simulink model "reaction_pendulum"  (R2021b)
settings: Solver=FixedStepDiscrete  StartTime=0.0  StopTime=140  FixedStep=h  RelTol=1e-3  EnableMultiTasking=on
PreLoadFcn:
  | warning('off','MATLAB:dispatcher:InexactMatch');
InitFcn:
  | hwinit
values from neighbouring files (symbols this model uses):
  h = 0.05    [Identified_system1_data.mat]    (also in Identified_system2_data.mat; Identified_system3_data.mat; Identified_system4_data.mat; MotorID_data.mat)
  K = Synth_LQR(sys, "Greybox")    [A1masterMain.m]    (also in Controller_LQR.mat = [-0.0224541453394 1.5413407747e-07 0.00117109816368 -2.28642; kalman.m = P_1 * H'/(H*P_1*H' + R))
  K_Unst = Synth_LQR(sysUnst, "Greybox")    [A1masterMain.m]
  params = cell2struct([struct2cell(motorparams);struct2cell(pendparams)],[fieldnames(motorparams);fieldnames(pendparams)],1)    [A1masterMain_Measurements.m]
  sys = ss(sys.A, sys.B, eye(nx), zeros(nx,1), h)    [A1masterMain.m]    (also in A1masterMain_Measurements.m; SysIDgrey_fullParamed.m = ss(Ac,Bc,Cc,Dc); SysIDgrey_motor.m = ss(Ac,Bc,Cc,Dc); SysIDgrey_semiParamed.m = ss(Ac,Bc,Cc,Dc))
undefined symbols (not defined in the file or in its folder): DiscIntNeverNeededParam, Discrete, Hinf, HinfI, HinfUnst, HinfUnstI, Ki, Ki_Unst, sysObserver, Time
libraries: simulink x5, mpclib x5, eeGeneralControl x2, ctrlSharedLib x2, sharedTrackingLibrary x1, eeLuenbergerObserver x1, pid_lib x1
settings Model: SimulationMode=external  ExtModeTrigDuration=100000  Creator=user  LastModifiedBy=saumans
settings DataIOCC: SaveFormat=Array  SignalLoggingSaveFormat=ModelDataLogs  SaveOutput=off  SignalLogging=off  DSMLogging=off  SaveTime=off  ReturnWorkspaceOutputs=off
settings OptimizationCC: ExpressionDepthLimit=2147483647  LifeSpan=inf
settings DebuggingCC: UnderspecifiedInitializationDetection=Classic  MergeDetectMultiDrivingBlocksExec=none  SolverPrmCheckMsg=warning  FcnCallInpInsideContextMsg=warning  StateNameClashWarn=warning  SFUnexpectedBacktrackingDiag=warning  SFNoUnconditionalDefaultTransitionDiag=warning  SFExecutionAtInitializationDiag=none  SFMachineParentedDataDiag=warning  ArithmeticOperatorsInVariantConditions=warning
settings HardwareCC: ProdBitPerPointer=32  ProdBitPerSizeT=32  ProdBitPerPtrDiffT=32  ProdLargestAtomicFloat=None  ProdIntDivRoundTo=Undefined  ProdEndianess=Unspecified  ProdWordSize=32  ProdHWDeviceType=32-bit Generic
settings ModelReferenceCC: PropagateSignalLabelsOutOfModel=off
settings SFSimCC: SimUseLocalCustomCode=off  CustomCodeUndefinedFunction=UseInterfaceOnly
settings RTWCC: Description=rpend RTDAC/USB2 (Visual C/C++)  SystemTargetFile=rtcon_rpend_usb2.tlc  TemplateMakefile=rtcon_rpend_vc_usb2_x64.tmf  RTWUseLocalCustomCode=off
settings CodeAppCC: StateflowObjectComments=on
settings STFCustomTargetCC: ModelReferenceCompliant=off  CombineOutputUpdateFcns=on  MatFileLogging=on  GRTInterface=off  SystemTargetFile=rtcon_rpend_usb2.tlc
settings GRTTargetCC: TargetLangStandard=C89/C90 (ANSI)  ModelReferenceCompliant=off  ParMdlRefBuildCompliant=off  CompOptLevelCompliant=off  ConcurrentExecutionCompliant=off  CPPClassGenCompliant=off  UseToolchainInfoCompliant=off  ExtMode=on  ExtModeMexFile=rtcon_ext_comm
settings ConfigComp: CovMetricSettings=dw  CovSaveCumulativeToWorkspaceVar=on  CovSaveSingleToWorkspaceVar=on  CovExternalEMLEnable=off  CovSFcnEnable=off

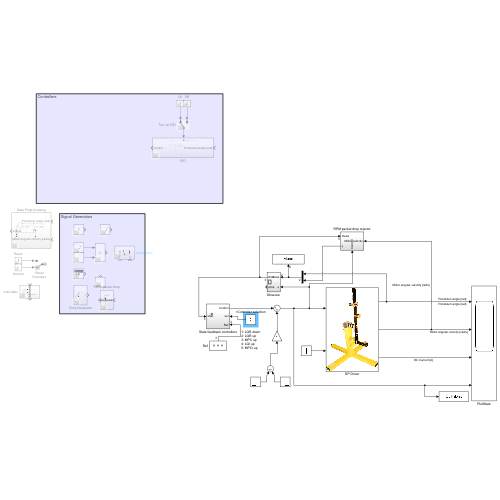
[thumbnail: Simulink's stored preview of the top-level diagram]
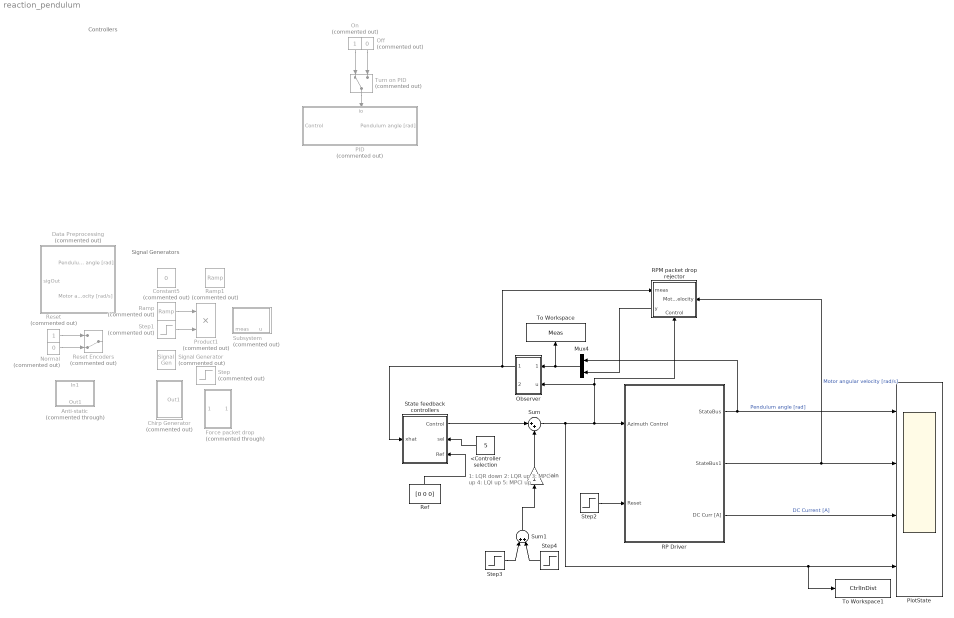
== system reaction_pendulum ==
  note: 1: LQR down
      | 2: LQR up
      | 3: MPC up
      | 4: LQI up
      | 5: MPCI up
  note: Controllers
  note: Signal Generators
  <Controller selection : Constant  Value=5
  Anti-static : Subsystem  Commented=through
  Chirp Generator : Subsystem  Commented=on
  Constant5 : Constant  Commented=on  Value=0
  Data Preprocessing : Subsystem  Commented=on
  Force packet drop : Subsystem  Commented=through
  Gain : Gain
  Mux4 : Mux  Inputs=2
  Normal : Constant  Commented=on  Value=0
  Observer : Subsystem
  Off : Constant  Commented=on  Value=0
  On : Constant  Commented=on
  PID : Subsystem  Commented=on
      settings: PortSchema="{\"entries\":[{\"content\":{\"sides\":[{\"content\":{\"connectorIds\":[\"In1\"]},\"type\":\"ConnectorPlacement.EquallySpacedRectSide\",\"uuid\":\"f2fec2e3-226e-4957-a417-0defdc291ba5\"},{\"content\":{\"connectorIds\":[\"Out1\"],\"side\":\"RIGHT\"},\"type\":\"ConnectorPlacement.EquallySpacedRectSide\",\"uuid\":\"376d4e87-61ea-4bcd-a986-cfc18b67c5cf\"},{\"content\":{\"connectorIds\":[\"In2\"],\"side\":\"TOP\"},\"type\":\"ConnectorPlacement.EquallySpacedRectSide\",\"uuid\":\"5745c80a-bb5a-4df3-811e-7eecb0205f19\"}]},\"type\":\"ConnectorPlacement.EquallySpacedConnector\",\"uuid\":\"e1ac6d12-4a7f-4ceb-9bf6-49805cc7f347\"}],\"packageUris\":[\"http://schema.mathworks.com/mf0/Connector/R2020b\"],\"version\":\"1.0\"}"
  PlotState : Scope  NumInputPorts=4
  Product1 : Product  Commented=on
  RP Driver : Subsystem
      mask Display: image(imread('rwp.JPG'))
  RPM packet drop rejector : Subsystem
      settings: PortSchema="{\"entries\":[{\"content\":{\"sides\":[{\"content\":{\"connectorIds\":[\"In1\"]},\"type\":\"ConnectorPlacement.EquallySpacedRectSide\",\"uuid\":\"dc71c52c-be7a-4309-9ef6-de56d2efa973\"},{\"content\":{\"connectorIds\":[\"In3\",\"Out1\"],\"side\":\"RIGHT\"},\"type\":\"ConnectorPlacement.EquallySpacedRectSide\",\"uuid\":\"4ea731d9-e83e-45db-852e-b55f70ff1dcb\"},{\"content\":{\"connectorIds\":[],\"side\":\"TOP\"},\"type\":\"ConnectorPlacement.EquallySpacedRectSide\",\"uuid\":\"11ed21a3-acf9-42d7-b1cb-d4047d3b6345\"},{\"content\":{\"connectorIds\":[\"In2\"],\"side\":\"BOTTOM\"},\"type\":\"ConnectorPlacement.EquallySpacedRectSide\",\"uuid\":\"19313e71-7ed6-479a-97a2-a24af120137a\"}]},\"type\":\"ConnectorPlacement.EquallySpacedConnector\",\"uuid\":\"3af8e27e-d2cb-4c9f-8435-3e2adc15d5d9\"}],\"packageUris\":[\"http://schema.mathworks.com/mf0/Connector/R2020b\"],\"version\":\"1.0\"}"
  Ramp : simulink/Sources/Ramp  Commented=on  slope=0.5/29  start=1  InitialOutput=0
  Ramp1 : simulink/Sources/Ramp  Commented=on  slope=0.5/29  start=1  InitialOutput=0
  Ref : Constant  Value=[0 0 0]
  Reset : Constant  Commented=on
  Reset Encoders : ManualSwitch  Commented=on  CurrentSetting=0
  Signal Generator : SignalGenerator  Commented=on  Amplitude=0.5  Frequency=0.1
  State feedback controllers : Subsystem
      settings: PortSchema="{\"entries\":[{\"content\":{\"sides\":[{\"content\":{\"connectorIds\":[\"In1\"]},\"type\":\"ConnectorPlacement.EquallySpacedRectSide\",\"uuid\":\"50f77728-1820-4c1e-b55e-992377a2ac74\"},{\"content\":{\"connectorIds\":[\"Out1\",\"In2\",\"In3\"],\"side\":\"RIGHT\"},\"type\":\"ConnectorPlacement.EquallySpacedRectSide\",\"uuid\":\"85e2483e-83dd-4c22-9320-33a68cb16c11\"},{\"content\":{\"connectorIds\":[],\"side\":\"TOP\"},\"type\":\"ConnectorPlacement.EquallySpacedRectSide\",\"uuid\":\"96f413ab-f651-4769-ae7d-08868bc0ab5d\"}]},\"type\":\"ConnectorPlacement.EquallySpacedConnector\",\"uuid\":\"cd5e282e-a58c-452a-9f76-0f6edfd53294\"}],\"packageUris\":[\"http://schema.mathworks.com/mf0/Connector/R2020b\"],\"version\":\"1.0\"}"
  Step : Step  Commented=on  Time=1.5  SampleTime=h
  Step1 : Step  Commented=on  Time=30  Before=1  After=0  SampleTime=h
  Step2 : Step  Time=h  Before=1  After=0  SampleTime=0
  Step3 : Step  Time=2  SampleTime=0
  Step4 : Step  Time=2.2  After=-1  SampleTime=0
  Subsystem : Subsystem  Commented=on
  Sum : Sum  Inputs=|++
  Sum1 : Sum  Inputs=|++|
  To Workspace : ToWorkspace  VariableName=Meas  SampleTime=h
      settings: Save2DSignal=2-D array (concatenate along first dimension)
  To Workspace1 : ToWorkspace  VariableName=CtrlInDist  SaveFormat=Structure With Time  SampleTime=h
      settings: Save2DSignal=2-D array (concatenate along first dimension)
  Turn on PID : ManualSwitch  Commented=on
  wires:
  Normal/1 -> Reset Encoders/2
  Reset/1 -> Reset Encoders/1
  Step2/1 -> RP Driver/2(Reset)
  RP Driver/3(DC Curr [A]) -> PlotState/3  "DC Current [A]"
  RP Driver/2(StateBus1) -> RPM packet drop rejector/1(Motor velocity), PlotState/2  "Motor angular velocity [rad/s]"
  RP Driver/1(StateBus) -> PlotState/1, Mux4/1  "Pendulum angle [rad]"
  On/1 -> Turn on PID/1
  Off/1 -> Turn on PID/2
  Turn on PID/1 -> PID/2(io)
  Step1/1 -> Product1/2
  Ramp/1 -> Product1/1
  <Controller selection/1 -> State feedback controllers/2(sel)
  Ref/1 -> State feedback controllers/3(Ref)
  RPM packet drop rejector/1(y) -> Mux4/2
  Mux4/1 -> To Workspace/1, Observer/1(meas)
  Sum/1 -> To Workspace1/1, PlotState/4, RPM packet drop rejector/2(Control), Observer/2(u), RP Driver/1(Azimuth Control)
  Observer/1(xhat) -> State feedback controllers/1(xhat), RPM packet drop rejector/3(meas)
  State feedback controllers/1(Control) -> Sum/1
  Gain/1 -> Sum/2
  Sum1/1 -> Gain/1
  Step3/1 -> Sum1/1
  Step4/1 -> Sum1/2

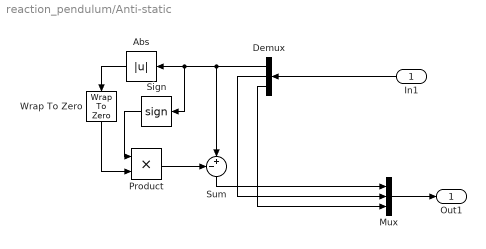
== system reaction_pendulum/Anti-static ==
  In1 : Inport
  Abs : Abs
  Demux : Demux  Outputs=3
  Mux : Mux  Inputs=3
  Product : Product
  Sign : Signum
  Sum : Sum  Inputs=-+|
  Wrap To Zero : simulink/Discontinuities/Wrap To Zero  Threshold=0.005
      settings: SourceProductBaseCode=SL
  Out1 : Outport
  wires:
  Demux/1 -> Sign/1, Abs/1, Sum/2
  Wrap To Zero/1 -> Product/2
  Sum/1 -> Mux/1
  Mux/1 -> Out1/1
  Sign/1 -> Product/1
  Product/1 -> Sum/1
  In1/1 -> Demux/1
  Abs/1 -> Wrap To Zero/1
  Demux/3 -> Mux/3
  Demux/2 -> Mux/2

== system reaction_pendulum/Chirp Generator ==
  Chirp Signal : simulink/Sources/Chirp Signal  f1=0.025  T=100  f2=0.75
  Gain3 : Gain  Gain=0.2
  Product3 : Product
  varMag_chirp_generator : Subsystem
  Out1 : Outport
  wires:
  Gain3/1 -> Out1/1
  Chirp Signal/1 -> Product3/1
  varMag_chirp_generator/1(Out1) -> Product3/2
  Product3/1 -> Gain3/1

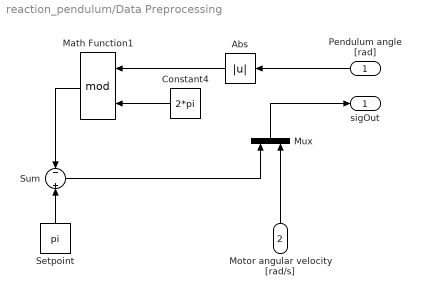
== system reaction_pendulum/Data Preprocessing ==
  Pendulum angle [rad] : Inport
  Motor angular velocity [rad/s] : Inport  Port=2
  Abs : Abs
  Constant4 : Constant  Value=2*pi
  Math Function1 : Math  Operator=mod  SaturateOnIntegerOverflow=on
  Mux : Mux  Inputs=2
  Setpoint : Constant  Value=pi
  Sum : Sum  Inputs=-||+
  sigOut : Outport
  wires:
  Motor angular velocity [rad/s]/1 -> Mux/2
  Sum/1 -> Mux/1
  Abs/1 -> Math Function1/1
  Math Function1/1 -> Sum/1
  Pendulum angle [rad]/1 -> Abs/1
  Setpoint/1 -> Sum/2
  Constant4/1 -> Math Function1/2
  Mux/1 -> sigOut/1

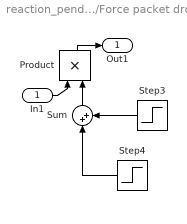
== system reaction_pendulum/Force packet drop ==
  In1 : Inport
  Product : Product
  Step3 : Step  Time=10+7*h  SampleTime=0
  Step4 : Step  Time=10  Before=1  After=0  SampleTime=0
  Sum : Sum  Inputs=|++
  Out1 : Outport
  wires:
  Step4/1 -> Sum/1
  Step3/1 -> Sum/2
  Product/1 -> Out1/1
  Sum/1 -> Product/2
  In1/1 -> Product/1

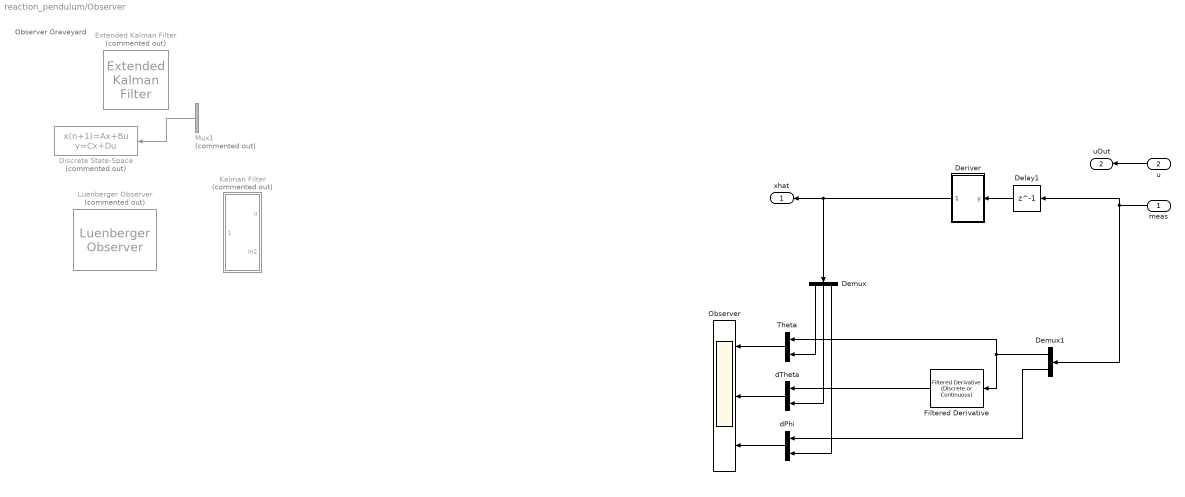
== system reaction_pendulum/Observer ==
  note: Observer Graveyard
  meas : Inport
  u : Inport  Port=2
  Delay1 : Delay  DelayLength=1  InitialCondition=0
  Demux : Demux  Outputs=3
  Demux1 : Demux  Outputs=2
  Deriver : Subsystem
  Discrete State-Space : DiscreteStateSpace  Commented=on  A=sysObserver.A  B=sysObserver.B  C=sysObserver.C  D=sysObserver.D  SampleTime=h
  Extended Kalman Filter : sharedTrackingLibrary/Extended Kalman Filter  Commented=on  StateTransitionFcn=nextIter  HasStateTransitionJacobianFcn=off  HasAdditiveProcessNoise=Additive  ProcessNoise=1  HasTimeVaryingProcessNoise=off  HasStateTransitionFcnExtraArgument=0  InitialState=0  InitialStateCovariance=1  MeasurementFcn1=myMeasurementFcn  HasMeasurementJacobianFcn1=off  HasMeasurementEnablePort1=off  HasAdditiveMeasurementNoise1=Additive  MeasurementNoise1=1  HasTimeVaryingMeasurementNoise1=off  HasMeasurementFcnExtraArgument1=0  MeasurementFcn2=myMeasurementFcn  HasMeasurementJacobianFcn2=off  HasMeasurementEnablePort2=off  HasAdditiveMeasurementNoise2=Additive  MeasurementNoise2=1  HasTimeVaryingMeasurementNoise2=off  HasMeasurementFcnExtraArgument2=0  MeasurementFcn3=myMeasurementFcn  HasMeasurementJacobianFcn3=off  HasMeasurementEnablePort3=off  HasAdditiveMeasurementNoise3=Additive  MeasurementNoise3=1  HasTimeVaryingMeasurementNoise3=off  HasMeasurementFcnExtraArgument3=0  MeasurementFcn4=myMeasurementFcn  HasMeasurementJacobianFcn4=off  HasMeasurementEnablePort4=off  HasAdditiveMeasurementNoise4=Additive  MeasurementNoise4=1  HasTimeVaryingMeasurementNoise4=off  HasMeasurementFcnExtraArgument4=0  MeasurementFcn5=myMeasurementFcn  HasMeasurementJacobianFcn5=off  HasMeasurementEnablePort5=off  HasAdditiveMeasurementNoise5=Additive  MeasurementNoise5=1  HasTimeVaryingMeasurementNoise5=off  HasMeasurementFcnExtraArgument5=0  EnableMultirate=off  StateTransitionFcnSampleTime=1  MeasurementFcn1SampleTime=1  MeasurementFcn2SampleTime=1  MeasurementFcn3SampleTime=1  MeasurementFcn4SampleTime=1  MeasurementFcn5SampleTime=1  UseCurrentEstimator=on  OutputStateCovariance=off  DataType=double  SampleTime=1  NumberOfMeasurements=1
      settings: SourceProductBaseCode=AE,PW,CT,DR,TF,ID,LP,NV,AR,RO,RR,UV,VE
  Filtered Derivative : eeGeneralControl/Filtered Derivative (Discrete or Continuous)  K=1  T=h  B=inf  A=-inf  minRatio=1  init_option=Specify as parameter  x0=0  Ts=h
      settings: SourceProductBaseCode=PS
  Kalman Filter : Subsystem  Commented=on
  Luenberger Observer : eeLuenbergerObserver/Luenberger Observer  Commented=on  StateSpaceType=Discrete-time  Ad=sys.A  Bd=sys.B  Cd=sys.C  Dd=sys.D  A=1  B=1  C=1  D=1  ObserverDesign=Desired eigenvalues  Ld=1  DesiredEigenvalues=0.2+(1:size(sys.A, 2))*0.001  x0=zeros(size(sys.A, 2), 1)  Tsd=0.1  Ts=h
      settings: SourceProductBaseCode=PS
  Mux1 : Mux  Commented=on  Inputs=2
  Observer : Scope  NumInputPorts=3
  Theta : Mux  Inputs=2
  dPhi : Mux  Inputs=2
  dTheta : Mux  Inputs=2
  xhat : Outport
  uOut : Outport  Port=2
  wires:
  meas/1 -> Demux1/1, Delay1/1
  Deriver/1(xhat) -> Demux/1, xhat/1
  Mux1/1 -> Discrete State-Space/1
  Theta/1 -> Observer/1
  dTheta/1 -> Observer/2
  dPhi/1 -> Observer/3
  Filtered Derivative/1 -> dTheta/1
  Demux/1 -> Theta/2
  Demux/2 -> dTheta/2
  Demux/3 -> dPhi/2
  Demux1/1 -> Theta/1, Filtered Derivative/1
  Demux1/2 -> dPhi/1
  u/1 -> uOut/1
  Delay1/1 -> Deriver/1(y)

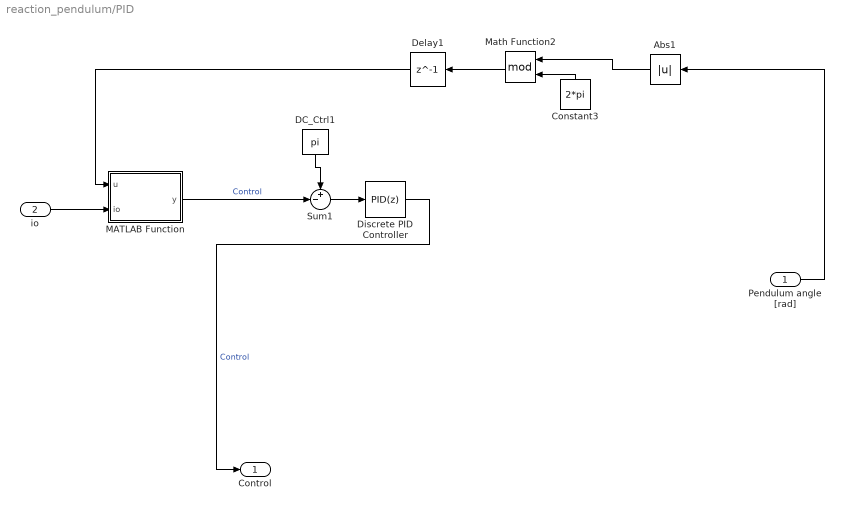
== system reaction_pendulum/PID ==
  Pendulum angle [rad] : Inport
  io : Inport  Port=2
  Abs1 : Abs
  Constant3 : Constant  Value=2*pi
  DC_Ctrl1 : Constant  Value=pi
  Delay1 : Delay  DelayLength=1  InitialCondition=0
  Discrete PID Controller : pid_lib/PID Controller  Controller=PID  Form=Parallel  TimeDomain=Discrete-time  UseExternalTs=off  SampleTime=h  IntegratorMethod=Forward Euler  FilterMethod=Forward Euler  ControllerParametersSource=internal  P=5.451713395638629  I=2.984615384615385  D=2.369230769230769  N=3  UseFilter=on  TunerSelectOption=Frequency Response Based  InitialConditionSource=internal  InitialConditionForIntegrator=0  InitialConditionForFilter=0  DifferentiatorICPrevScaledInput=0  ExternalReset=none  TrackingMode=off  Kt=1  LimitOutput=off  SatLimitsSource=internal  UpperSaturationLimit=inf  LowerSaturationLimit=-inf  LinearizeAsGain=off  AntiWindupMode=none  Kb=1  POutMin=[]  POutMax=[]  IOutMin=[]  IOutMax=[]  DOutMin=[]  DOutMax=[]  NOutMin=[]  NOutMax=[]  SumOutMin=[]  SumOutMax=[]  SaturationOutMin=[]  SaturationOutMax=[]  PParamMin=[]  PParamMax=[]  IParamMin=[]  IParamMax=[]  DParamMin=[]  DParamMax=[]  NParamMin=[]  NParamMax=[]  KbParamMin=[]  KbParamMax=[]  KtParamMin=[]  KtParamMax=[]  KbOutMin=[]  KbOutMax=[]  KtOutMin=[]  KtOutMax=[]  IntegratorOutMin=[]  IntegratorOutMax=[]  FilterOutMin=[]  FilterOutMax=[]  SumI1OutMin=[]  SumI1OutMax=[]  SumI2OutMin=[]  SumI2OutMax=[]  SumI3OutMin=[]  SumI3OutMax=[]  SumI4OutMin=[]  SumI4OutMax=[]  SumDOutMin=[]  SumDOutMax=[]  DifferentiatorOutMin=[]  DifferentiatorOutMax=[]  FilterDiffOutCoefMin=[]  FilterDiffOutCoefMax=[]  ReciprocalOutMin=[]  ReciprocalOutMax=[]  SumDenOutMin=[]  SumDenOutMax=[]  SumNumOutMin=[]  SumNumOutMax=[]  DivideOutMin=[]  DivideOutMax=[]  UdiffTsProdOutMin=[]  UdiffTsProdOutMax=[]  NTsProdOutMin=[]  NTsProdOutMax=[]  UintegralTsProdOutMin=[]  UintegralTsProdOutMax=[]  UngainTsProdOutMin=[]  UngainTsProdOutMax=[]  IntegratorContinuousStateAttributes=''  IntegratorStateMustResolveToSignalObject=off  IntegratorRTWStateStorageClass=Auto  FilterContinuousStateAttributes=''  FilterStateMustResolveToSignalObject=off  FilterRTWStateStorageClass=Auto  ParallelPVariant=InternalParameters  IdealPVariant=Disabled  IVariant=InternalParameters  DVariant=InternalParameters  IntegratorVariant=Discrete  SatVariant=Disabled  AWVariant=Passthrough  PCopyVariant=Disabled  TRVariant=Disabled  FdbkBlocksVariant=Forward  IdealPFdbkVariant=Disabled  SatFdbkVariant=Disabled  DerivativeFilterVariant=ForwardEulerFilter  NVariant=InternalParameters  NCopyVariant=Disabled  FilterICVariant=InternalICsFilter  IntegratorICVariant=InternalICs  ExternalResetVariant=Disabled  TRSumVariant=Passthrough  SumFdbkVariant=Disabled  SumVariant=Sum_PID  TsampFilterVariant=InternalTs  TsampNgainVariant=Passthrough  TsampIntegralVariant=Passthrough  ExternalSaturationOutDataTypeStr=Inherit: Same as second input
  MATLAB Function : MATLAB Function  TreatAsAtomicUnit=on
  Math Function2 : Math  Operator=mod  SaturateOnIntegerOverflow=on
  Sum1 : Sum  Inputs=+-|
  Control : Outport
  wires:
  Constant3/1 -> Math Function2/2
  Math Function2/1 -> Delay1/1
  Sum1/1 -> Discrete PID Controller/1
  Abs1/1 -> Math Function2/1
  Discrete PID Controller/1 -> Control/1  "Control"
  Delay1/1 -> MATLAB Function/1(u)
  MATLAB Function/1(y) -> Sum1/2  "Control"
  DC_Ctrl1/1 -> Sum1/1
  Pendulum angle [rad]/1 -> Abs1/1
  io/1 -> MATLAB Function/2(io)

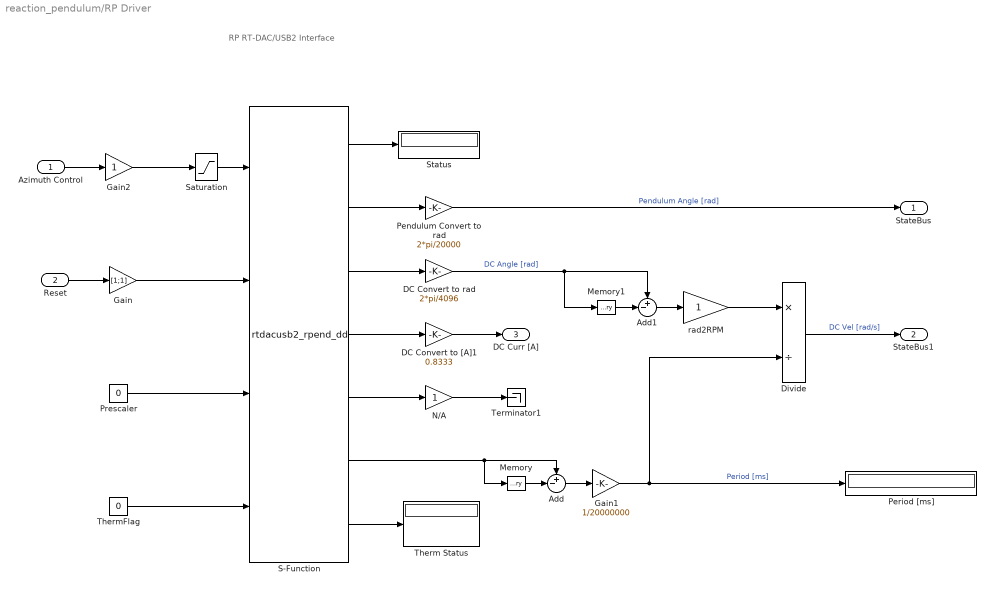
== system reaction_pendulum/RP Driver ==
  note: RP RT-DAC/USB2
      | Interface
  Azimuth Control : Inport
  Reset : Inport  Port=2
  Add : Sum  Inputs=+-|
  Add1 : Sum  Inputs=+-|
  DC Convert to [A]1 : Gain  Gain=0.8333  SaturateOnIntegerOverflow=on  OutDataTypeStr=Inherit: Same as input  ParamDataTypeStr=Inherit: Same as input
  DC Convert to rad : Gain  Gain=2*pi/4096  SaturateOnIntegerOverflow=on  OutDataTypeStr=Inherit: Same as input  ParamDataTypeStr=Inherit: Same as input
  Divide : Product  Inputs=*/
  Gain : Gain  Gain=[1;1]
  Gain1 : Gain  Gain=1/20000000
  Gain2 : Gain
  Memory : Memory
  Memory1 : Memory
  N/A : Gain  SaturateOnIntegerOverflow=on  OutDataTypeStr=Inherit: Same as input  ParamDataTypeStr=Inherit: Same as input
  Pendulum Convert to rad : Gain  Gain=2*pi/20000  SaturateOnIntegerOverflow=on  OutDataTypeStr=Inherit: Same as input  ParamDataTypeStr=Inherit: Same as input
  Period [ms] : Display
  Prescaler : Constant  Value=0
  S-Function : S-Function  FunctionName=rtdacusb2_rpend_dd  Parameters=1, h  SFunctionDeploymentMode=off  EnableBusSupport=off
  Saturation : Saturate  UpperLimit=1  LowerLimit=-1
  Status : Display
  Terminator1 : Terminator
  Therm Status : Display
  ThermFlag : Constant  Value=0
  rad2RPM : Gain  SaturateOnIntegerOverflow=on  OutDataTypeStr=Inherit: Same as input  ParamDataTypeStr=Inherit: Same as input
  StateBus : Outport  VectorParamsAs1DForOutWhenUnconnected=off
  StateBus1 : Outport  Port=2  VectorParamsAs1DForOutWhenUnconnected=off
  DC Curr [A] : Outport  Port=3  VectorParamsAs1DForOutWhenUnconnected=off
  wires:
  S-Function/7 -> Therm Status/1
  S-Function/5 -> N/A/1
  S-Function/4 -> DC Convert to [A]1/1
  ThermFlag/1 -> S-Function/4
  Prescaler/1 -> S-Function/3
  Gain/1 -> S-Function/2
  DC Convert to [A]1/1 -> DC Curr [A]/1
  Divide/1 -> StateBus1/1  "DC Vel [rad/s]"
  rad2RPM/1 -> Divide/1
  Add1/1 -> rad2RPM/1
  Memory1/1 -> Add1/2
  N/A/1 -> Terminator1/1
  S-Function/6 -> Add/1, Memory/1
  Gain2/1 -> Saturation/1
  Gain1/1 -> Period [ms]/1, Divide/2  "Period [ms]"
  Add/1 -> Gain1/1
  Memory/1 -> Add/2
  DC Convert to rad/1 -> Add1/1, Memory1/1  "DC Angle [rad]"
  S-Function/3 -> DC Convert to rad/1
  Pendulum Convert to rad/1 -> StateBus/1  "Pendulum Angle [rad]"
  S-Function/2 -> Pendulum Convert to rad/1
  S-Function/1 -> Status/1
  Saturation/1 -> S-Function/1
  Reset/1 -> Gain/1
  Azimuth Control/1 -> Gain2/1

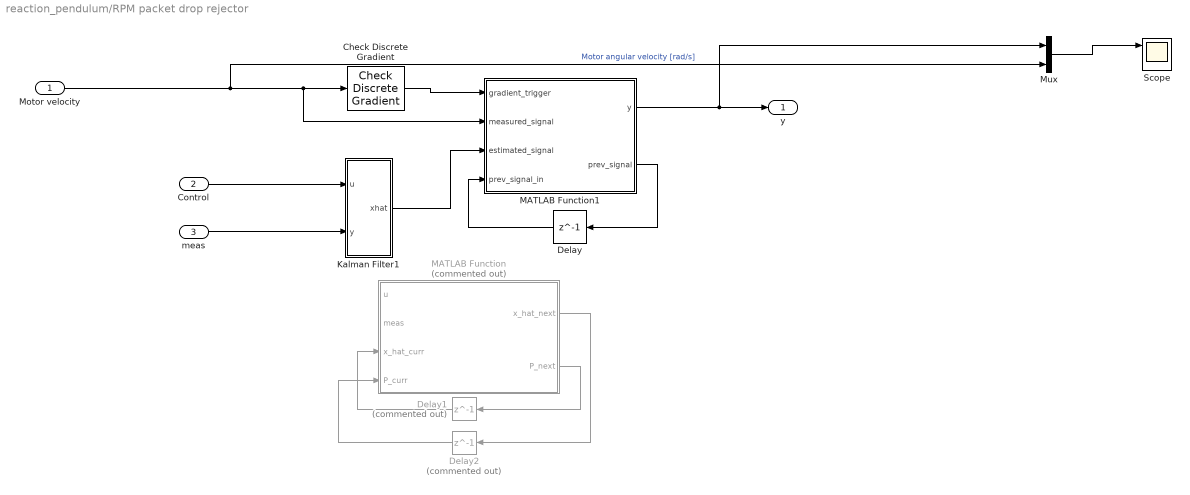
== system reaction_pendulum/RPM packet drop rejector ==
  Motor velocity : Inport
  Control : Inport  Port=2
  meas : Inport  Port=3
  Check Discrete Gradient : simulink/Model Verification/Check Discrete Gradient  Description=| du / dt | < 50  gradient=50  enabled=on  stopWhenAssertionFail=off  export=on  icon=graphic
      settings: SourceProductBaseCode=SL
  Delay : Delay  DelayLength=1  InitialCondition=0
  Delay1 : Delay  Commented=on  DelayLength=1
  Delay2 : Delay  Commented=on  DelayLength=1
  Kalman Filter1 : Subsystem
  MATLAB Function : MATLAB Function  Commented=on  TreatAsAtomicUnit=on
  MATLAB Function1 : MATLAB Function  TreatAsAtomicUnit=on
  Mux : Mux  Inputs=2
  Scope : Scope  NumInputPorts=3
  y : Outport
  wires:
  Check Discrete Gradient/1 -> MATLAB Function1/1(gradient_trigger)
  Kalman Filter1/1(xhat) -> MATLAB Function1/3(estimated_signal)
  Control/1 -> Kalman Filter1/1(u)
  MATLAB Function1/2(prev_signal) -> Delay/1
  Delay/1 -> MATLAB Function1/4(prev_signal_in)
  Motor velocity/1 -> Mux/2, MATLAB Function1/2(measured_signal), Check Discrete Gradient/1  "Motor angular velocity [rad/s]"
  MATLAB Function1/1(y) -> Mux/1, y/1
  Mux/1 -> Scope/1
  meas/1 -> Kalman Filter1/2(y)
  MATLAB Function/2(P_next) -> Delay1/1
  Delay1/1 -> MATLAB Function/3(x_hat_curr)
  MATLAB Function/1(x_hat_next) -> Delay2/1
  Delay2/1 -> MATLAB Function/4(P_curr)

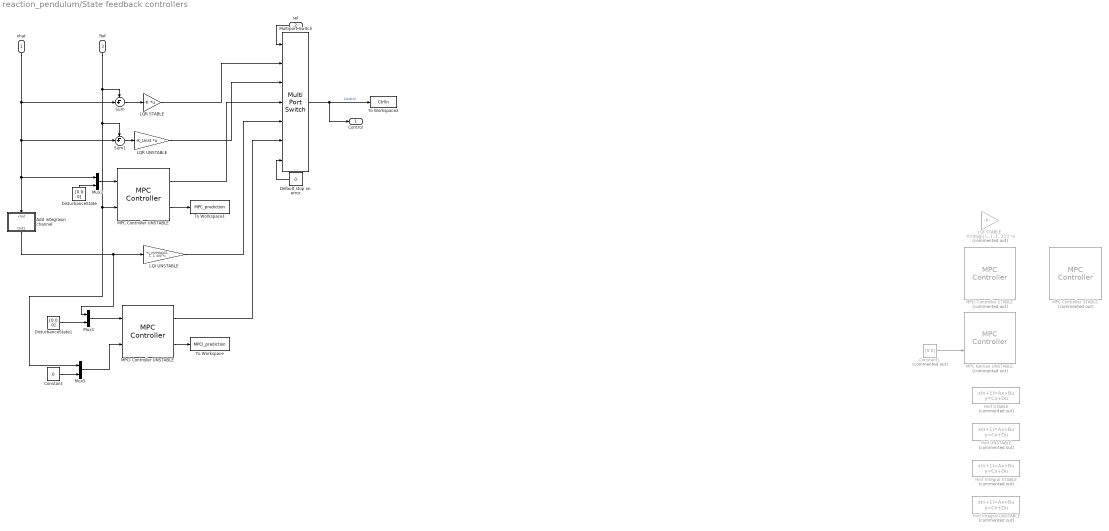
== system reaction_pendulum/State feedback controllers ==
  xhat : Inport
  sel : Inport  Port=2
  Ref : Inport  Port=3
  Add integraion channel : Subsystem
  Constant : Constant  Value=0
  Constant1 : Constant  Commented=on  Value=[0 0]
  Default stop on error : Constant  Value=0
  DisturbanceState : Constant  Value=[0 0 0]
  DisturbanceState1 : Constant  Value=[0 0 0]
  Hinf Integral STABLE : DiscreteStateSpace  Commented=on  A=HinfI.A  B=HinfI.B  C=HinfI.C  D=HinfI.D  SampleTime=-1
  Hinf Integral UNSTABLE : DiscreteStateSpace  Commented=on  A=HinfUnstI.A  B=HinfUnstI.B  C=HinfUnstI.C  D=HinfUnstI.D  SampleTime=-1
  Hinf STABLE : DiscreteStateSpace  Commented=on  A=Hinf.A  B=Hinf.B  C=Hinf.C  D=Hinf.D  SampleTime=-1
  Hinf UNSTABLE : DiscreteStateSpace  Commented=on  A=HinfUnst.A  B=HinfUnst.B  C=HinfUnst.C  D=HinfUnst.D  SampleTime=-1
  LQI STABLE : Gain  Commented=on  Gain=-Ki*diag([1, 1, 1, 35])  Multiplication=Matrix(K*u)
  LQI UNSTABLE : Gain  Gain=-Ki_Unst*diag([1, 1, 1, 40])  Multiplication=Matrix(K*u)
  LQR STABLE : Gain  Gain=-K  Multiplication=Matrix(K*u)
  LQR UNSTABLE : Gain  Gain=-K_Unst  Multiplication=Matrix(K*u)
  MPC Controller STABLE : mpclib/MPC Controller  Commented=on  SCDEnableBlockLinearizationSpecification=on  mpcobj=mpcController  is_multiple=0  enable_value=0  return_u0=off  updateMPCinCallerWorkspace=on  md_inport=off  mv_inport=off  uref_inport=off  return_cost=off  return_mvseq=off  return_qpstatus=off  return_xseq=off  return_state=off  return_ovseq=on  state_inport=on  umin_inport=off  umax_inport=off  ymin_inport=off  ymax_inport=off  cc_inport=off  ywt_inport=off  uwt_inport=off  duwt_inport=off  rhoeps_inport=off  pm_inport=off  MaximumP=10  HorizonChoice=FixedHorizon  n_ts=0.05  n_p=15  n_mv=1  n_md=0  n_ud=0  n_mo=3  n_uo=0  BlockDataType=double  SampleTimeInherited=off  switch_inport=off
  MPC Controller UNSTABLE : mpclib/MPC Controller  SCDEnableBlockLinearizationSpecification=on  mpcobj=mpcControllerUnst  is_multiple=0  enable_value=0  return_u0=off  updateMPCinCallerWorkspace=on  md_inport=off  mv_inport=off  uref_inport=off  return_cost=off  return_mvseq=off  return_qpstatus=off  return_xseq=off  return_state=off  return_ovseq=on  state_inport=on  umin_inport=off  umax_inport=off  ymin_inport=off  ymax_inport=off  cc_inport=off  ywt_inport=off  uwt_inport=off  duwt_inport=off  rhoeps_inport=off  pm_inport=off  MaximumP=10  HorizonChoice=FixedHorizon  n_ts=0.05  n_p=20  n_mv=1  n_md=0  n_ud=0  n_mo=3  n_uo=0  BlockDataType=double  SampleTimeInherited=off  switch_inport=off
  MPC kalman UNSTABLE : mpclib/MPC Controller  Commented=on  SCDEnableBlockLinearizationSpecification=on  mpcobj=mpcKalmanUnst  is_multiple=0  enable_value=0  return_u0=off  updateMPCinCallerWorkspace=on  md_inport=off  mv_inport=off  uref_inport=off  return_cost=off  return_mvseq=off  return_qpstatus=off  return_xseq=off  return_state=off  return_ovseq=on  state_inport=off  umin_inport=off  umax_inport=off  ymin_inport=off  ymax_inport=off  cc_inport=off  ywt_inport=off  uwt_inport=off  duwt_inport=off  rhoeps_inport=off  pm_inport=off  MaximumP=10  HorizonChoice=FixedHorizon  n_ts=0.05  n_p=10  n_mv=1  n_md=0  n_ud=0  n_mo=2  n_uo=0  BlockDataType=double  SampleTimeInherited=off  switch_inport=off
  MPCI Controller STABLE : mpclib/MPC Controller  Commented=on  SCDEnableBlockLinearizationSpecification=on  mpcobj=mpcI  is_multiple=0  enable_value=0  return_u0=off  updateMPCinCallerWorkspace=on  md_inport=off  mv_inport=off  uref_inport=off  return_cost=off  return_mvseq=off  return_qpstatus=off  return_xseq=off  return_state=off  return_ovseq=off  state_inport=on  umin_inport=off  umax_inport=off  ymin_inport=off  ymax_inport=off  cc_inport=off  ywt_inport=off  uwt_inport=off  duwt_inport=off  rhoeps_inport=off  pm_inport=off  MaximumP=10  HorizonChoice=FixedHorizon  n_ts=0.05  n_p=10  n_mv=1  n_md=0  n_ud=0  n_mo=4  n_uo=0  BlockDataType=double  SampleTimeInherited=off  switch_inport=off
  MPCI Controller UNSTABLE : mpclib/MPC Controller  SCDEnableBlockLinearizationSpecification=on  mpcobj=mpcIUnst  is_multiple=0  enable_value=0  return_u0=off  updateMPCinCallerWorkspace=on  md_inport=off  mv_inport=off  uref_inport=off  return_cost=off  return_mvseq=off  return_qpstatus=off  return_xseq=off  return_state=off  return_ovseq=on  state_inport=on  umin_inport=off  umax_inport=off  ymin_inport=off  ymax_inport=off  cc_inport=off  ywt_inport=off  uwt_inport=off  duwt_inport=off  rhoeps_inport=off  pm_inport=off  MaximumP=10  HorizonChoice=FixedHorizon  n_ts=0.05  n_p=20  n_mv=1  n_md=0  n_ud=0  n_mo=4  n_uo=0  BlockDataType=double  SampleTimeInherited=off  switch_inport=off
  Multiport Switch : MultiPortSwitch  Inputs=6
  Mux1 : Mux  Inputs=2
  Mux3 : Mux  Inputs=2
  Mux5 : Mux  Inputs=2
  Sum : Sum  Inputs=-+|
  Sum1 : Sum  Inputs=-+|
  To Workspace : ToWorkspace  VariableName=MPCI_prediction  SampleTime=-1
  To Workspace1 : ToWorkspace  VariableName=MPC_prediction  SampleTime=-1
  To Workspace2 : ToWorkspace  VariableName=CtrlIn  SaveFormat=Structure With Time  SampleTime=h
      settings: Save2DSignal=2-D array (concatenate along first dimension)
  Control : Outport
  wires:
  Multiport Switch/1 -> To Workspace2/1, Control/1  "Control"
  sel/1 -> Multiport Switch/1
  Sum/1 -> LQR STABLE/1
  Sum1/1 -> LQR UNSTABLE/1
  DisturbanceState/1 -> Mux3/2
  Mux3/1 -> MPC Controller UNSTABLE/1
  DisturbanceState1/1 -> Mux1/2
  Mux1/1 -> MPCI Controller UNSTABLE/1
  Ref/1 -> Sum/1, Sum1/1, Mux5/1, MPC Controller UNSTABLE/2
  Constant/1 -> Mux5/2
  Mux5/1 -> MPCI Controller UNSTABLE/2
  Constant1/1 -> MPC kalman UNSTABLE/2
  MPCI Controller UNSTABLE/2 -> To Workspace/1
  Add integraion channel/1(Out1) -> Mux1/1, LQI UNSTABLE/1
  xhat/1 -> Add integraion channel/1(xhat), Mux3/1, Sum1/2, Sum/2
  LQR STABLE/1 -> Multiport Switch/2
  LQR UNSTABLE/1 -> Multiport Switch/3
  MPC Controller UNSTABLE/1 -> Multiport Switch/4
  LQI UNSTABLE/1 -> Multiport Switch/5
  MPCI Controller UNSTABLE/1 -> Multiport Switch/6
  Default stop on error/1 -> Multiport Switch/7
  MPC Controller UNSTABLE/2 -> To Workspace1/1

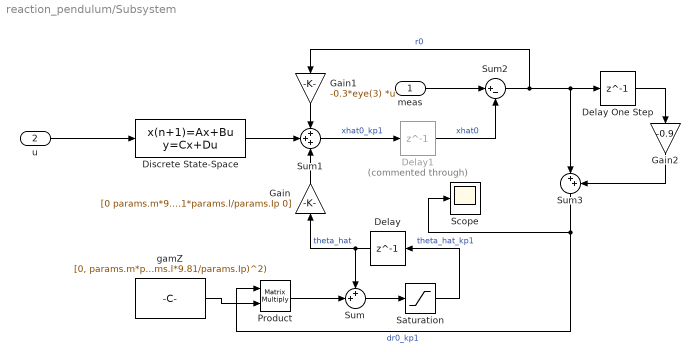
== system reaction_pendulum/Subsystem ==
  meas : Inport
  u : Inport  Port=2
  Delay : Delay  DelayLength=1  InitialCondition=0
  Delay One Step : Delay  DelayLength=1
  Delay1 : Delay  Commented=through  DelayLength=1  InitialCondition=0
  Discrete State-Space : DiscreteStateSpace  A=sys.A  B=sys.B  C=sys.C  D=sys.D  SampleTime=h
  Gain : Gain  Gain=[0 params.m*9.81*params.l/params.Ip 0]
  Gain1 : Gain  Gain=-0.3*eye(3)  Multiplication=Matrix(K*u)
  Gain2 : Gain  Gain=-0.9
  Product : Product  Multiplication=Matrix(*)
  Saturation : Saturate  UpperLimit=deg2rad(2)  LowerLimit=-deg2rad(2)
  Scope : Scope
  Sum : Sum  Inputs=++|
  Sum1 : Sum  Inputs=+++
  Sum2 : Sum  Inputs=|+-
  Sum3 : Sum  Inputs=|++
  gamZ : Constant  Value=[0, params.m*params.l*9.81/params.Ip, 0] .* 1/(1e-6 + abs(params.m*params.l*9.81/params.Ip)^2)
  wires:
  Delay1/1 -> Sum2/2  "xhat0"
  meas/1 -> Sum2/1
  Sum/1 -> Saturation/1
  Product/1 -> Sum/2
  Gain2/1 -> Sum3/2
  u/1 -> Discrete State-Space/1
  Sum1/1 -> Delay1/1  "xhat0_kp1"
  Saturation/1 -> Delay/1  "theta_hat_kp1"
  Discrete State-Space/1 -> Sum1/2
  Sum2/1 -> Gain1/1, Sum3/1, Delay One Step/1  "r0"
  Delay/1 -> Sum/1, Gain/1  "theta_hat"
  Gain/1 -> Sum1/3
  gamZ/1 -> Product/2
  Delay One Step/1 -> Gain2/1
  Gain1/1 -> Sum1/1
  Sum3/1 -> Product/1, Scope/1  "dr0_kp1"

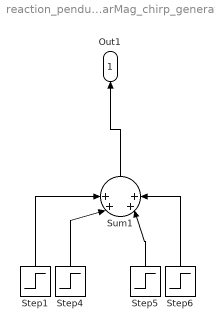
== system reaction_pendulum/Chirp Generator/varMag_chirp_generator ==
  Step1 : Step  Time=45  Before=1  After=0.3  SampleTime=h
  Step4 : Step  Time=50  After=0.7  SampleTime=h
  Step5 : Step  Time=60  After=-0.6  SampleTime=h
  Step6 : Step  Time=65  After=0  SampleTime=h
  Sum1 : Sum  Inputs=++|++
  Out1 : Outport
  wires:
  Sum1/1 -> Out1/1
  Step1/1 -> Sum1/1
  Step4/1 -> Sum1/2
  Step5/1 -> Sum1/3
  Step6/1 -> Sum1/4

== system reaction_pendulum/Observer/Deriver ==
  y : Inport
  Demux2 : Demux  Outputs=2
  Filtered Derivative1 : eeGeneralControl/Filtered Derivative (Discrete or Continuous)  K=1  T=h  B=inf  A=-inf  minRatio=1  init_option=Specify as parameter  x0=0  Ts=h
      settings: SourceProductBaseCode=PS
  Mux : Mux  Inputs=3
  xhat : Outport
  wires:
  Filtered Derivative1/1 -> Mux/2
  Demux2/1 -> Mux/1, Filtered Derivative1/1
  y/1 -> Demux2/1
  Demux2/2 -> Mux/3
  Mux/1 -> xhat/1

== system reaction_pendulum/Observer/Kalman Filter ==
  u : Inport
  In2 : Inport  Port=2
  Constant3 : Constant  Value=[0 0 0]  SampleTime=h
  Kalman Filter : ctrlSharedLib/Kalman Filter  TimeDomain=Discrete-Time  UseCurrentEstimator=on  ModelSource=LTI State-Space Variable  ModelSourceVariable=sys  A=0.95  B=1  C=1  D=0  NumberOfStates=1  NumberOfInputs=1  NumberOfOutputs=1  InitialEstimateSource=Input port  X0=0  P0=10  UseK=off  UseGH=off  NumberOfProcessNoiseInputs=1  G=1  TimeInvariantG=on  H=0  TimeInvariantH=on  Q=diag([1e-5 1e-2 1e-5])  TimeInvariantQ=on  R=1e-10*eye(size(sys.C,1))  TimeInvariantR=on  N=0  TimeInvariantN=on  AddInputPort=on  AddEnablePort=off  OutputEstimatedY=off  OutputP=off  Ts=-1
  Rate Transition : RateTransition  OutPortSampleTime=h
  xhat : Outport
  wires:
  In2/1 -> Rate Transition/1
  Rate Transition/1 -> Kalman Filter/2
  Constant3/1 -> Kalman Filter/3
  u/1 -> Kalman Filter/1
  Kalman Filter/1 -> xhat/1

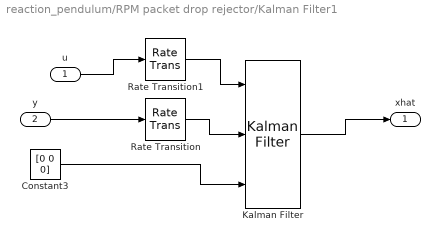
== system reaction_pendulum/RPM packet drop rejector/Kalman Filter1 ==
  u : Inport
  y : Inport  Port=2
  Constant3 : Constant  Value=[0 0 0]  SampleTime=h
  Kalman Filter : ctrlSharedLib/Kalman Filter  TimeDomain=Discrete-Time  UseCurrentEstimator=on  ModelSource=LTI State-Space Variable  ModelSourceVariable=sys  A=0.95  B=1  C=1  D=0  NumberOfStates=1  NumberOfInputs=1  NumberOfOutputs=1  InitialEstimateSource=Input port  X0=0  P0=10  UseK=off  UseGH=off  NumberOfProcessNoiseInputs=1  G=1  TimeInvariantG=on  H=0  TimeInvariantH=on  Q=diag([1e-5 1e-2 1e-5])  TimeInvariantQ=on  R=1e-10*eye(size(sys.C,1))  TimeInvariantR=on  N=0  TimeInvariantN=on  AddInputPort=on  AddEnablePort=off  OutputEstimatedY=off  OutputP=off  Ts=-1
  Rate Transition : RateTransition  OutPortSampleTime=h
  Rate Transition1 : RateTransition  OutPortSampleTime=h
  xhat : Outport
  wires:
  y/1 -> Rate Transition/1
  Rate Transition/1 -> Kalman Filter/2
  Constant3/1 -> Kalman Filter/3
  Kalman Filter/1 -> xhat/1
  u/1 -> Rate Transition1/1
  Rate Transition1/1 -> Kalman Filter/1

== system reaction_pendulum/State feedback controllers/Add integraion channel ==
  xhat : Inport
  Demux : Demux  Outputs=3
  Discrete-Time Integrator : DiscreteIntegrator  gainval=1  SampleTime=-1  ICPrevOutput=DiscIntNeverNeededParam  ICPrevScaledInput=DiscIntNeverNeededParam
  Mux : Mux
  To Workspace2 : ToWorkspace  VariableName=MeasFull  SampleTime=h
      settings: Save2DSignal=2-D array (concatenate along first dimension)
  Out1 : Outport
  wires:
  Mux/1 -> Out1/1, To Workspace2/1
  Demux/3 -> Mux/3
  Demux/2 -> Mux/2
  Demux/1 -> Discrete-Time Integrator/1, Mux/1
  Discrete-Time Integrator/1 -> Mux/4
  xhat/1 -> Demux/1

== matlab function reaction_pendulum/PID/MATLAB Function ==
  data: u input; y output; io input
function y = fcn(u, io)
if io == 1
    y = u;
else
    y = pi;
end
end

== matlab function reaction_pendulum/RPM packet drop rejector/MATLAB Function ==
  data: u input; x_hat_next output; meas input; x_hat_curr input; P_curr input; P_next output
function [x_hat_next,P_next] = fcn(u, meas,x_hat_curr,P_curr)

A = sys.A;
B = sys.B;
C = sys.C;
D = sys.D;
Q = diag([1e-5 1e-2 1e-5]);
R = 1e-10*eye(size(sys.C,1));


% if P_prev == 0
%     P = zeros(3,3);
% else
%     P = P_prev;
% end
% 
% if x_hat_curr == 0
%     x_hat_curr= [0 0 0];
% end




    
%     Time update
    x_hat_next = A*x_hat_curr';
    P_next = A*P_curr*A'+Q;        
%     Measurement update
    K = P_curr*C'/(C*P_curr*C'+R);
    x_hat_curr= x_hat_curr + (K*(-C*x_hat(k,:)'))';
    P_curr = P_curr - P_curr*C'/(C*P_curr*C'+R)*C*P_curr;       

end

== matlab function reaction_pendulum/RPM packet drop rejector/MATLAB Function1 ==
  data: gradient_trigger input; y output; measured_signal input; estimated_signal input; prev_signal_in input; prev_signal output
function [y, prev_signal] = fcn(gradient_trigger, measured_signal,estimated_signal, prev_signal_in)

    if(gradient_trigger == 1)        
        prev_signal = measured_signal;
    else
        prev_signal = 9999999;
    end

    if (prev_signal_in == measured_signal)
        y = estimated_signal(2);
    else
        y = measured_signal;
    end

end
